simulink model "OpenLoopStepResponse"  (R2024b)
settings: Solver=VariableStepAuto  StartTime=0.0  StopTime=10.0  RelTol=1e-3
settings Model: Creator=auw_a  LastModifiedBy=auw_a

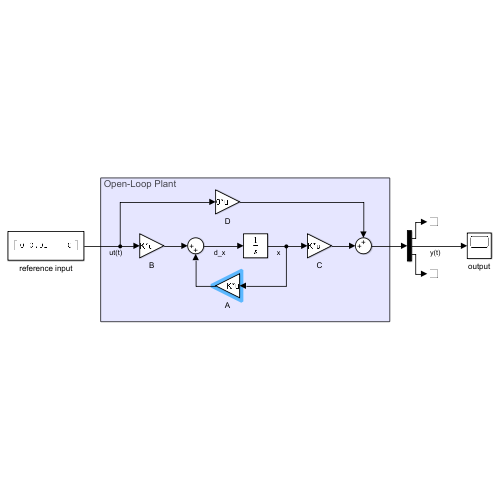
[thumbnail: Simulink's stored preview of the top-level diagram]
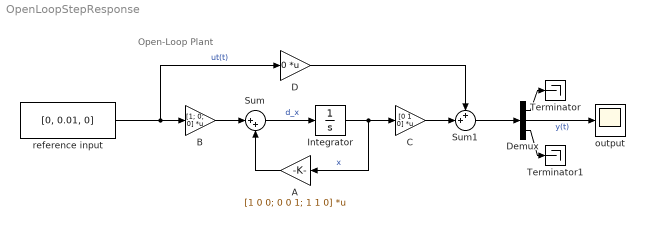
== system OpenLoopStepResponse ==
  note: Open-Loop Plant
  A : Gain  Gain=[1 0 0; 0 0 1; 1 1 0]  Multiplication=Matrix(K*u)
  B : Gain  Gain=[1; 0; 0]  Multiplication=Matrix(K*u)
  C : Gain  Gain=[0 1 0]  Multiplication=Matrix(K*u)
  D : Gain  Gain=0  Multiplication=Matrix(K*u)
  Demux : Demux  Outputs=3
  Integrator : Integrator
  Sum : Sum  Inputs=|++
  Sum1 : Sum  Inputs=++|
  Terminator : Terminator
  Terminator1 : Terminator
  output : Scope
  reference input : Constant  Value=[0, 0.01, 0]  VectorParams1D=off
  wires:
  B/1 -> Sum/1
  A/1 -> Sum/2
  Sum/1 -> Integrator/1  "d_x"
  Integrator/1 -> A/1, C/1  "x"
  C/1 -> Sum1/2
  D/1 -> Sum1/1
  reference input/1 -> D/1, B/1  "ut(t)"
  Sum1/1 -> Demux/1
  Demux/1 -> Terminator/1
  Demux/2 -> output/1  "y(t)"
  Demux/3 -> Terminator1/1
